simulink model "FDIA_Toolbox"  (R2018a)
settings: Solver=VariableStepAuto  StartTime=0.0  StopTime=10.0  RelTol=1e-3
libraries: commrandsrc3 x30, commutil2 x12, simulink_extras x6, simulink x4, commsynccomp2 x2, commanapbnd3 x2
(part 1 of 2)
settings Model: Creator=sasanka  LastModifiedBy=sasanka

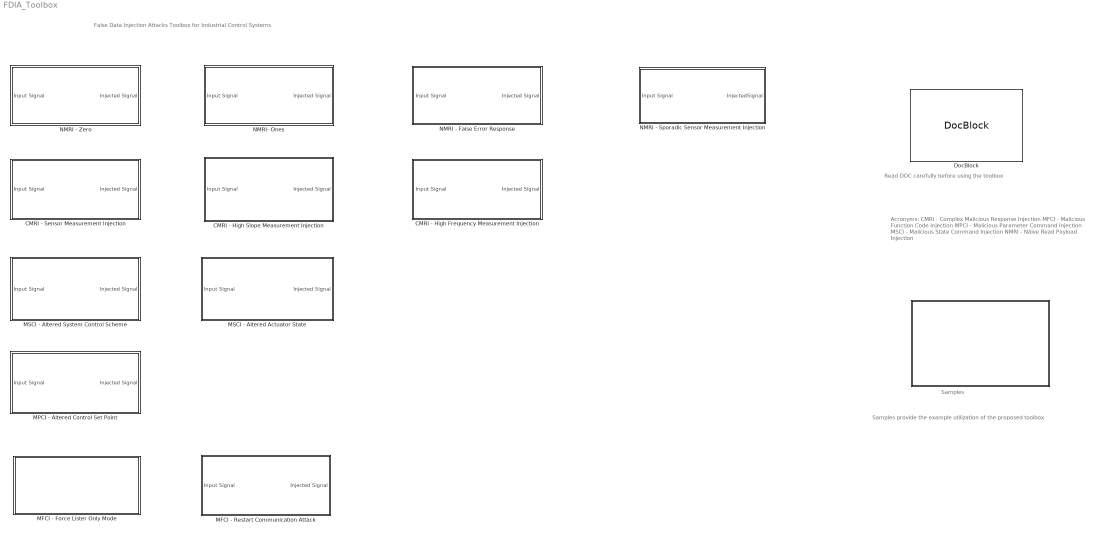
== system FDIA_Toolbox ==
  note: Samples provide the example utilization of the proposed toolbox
  note: Read DOC carefully before using the toolbox
  note: Acronyms:
      |
      | CMRI - Complex Malicious Response Injection
      | MFCI - Malicious Function Code Injection
      | MPCI - Malicious Parameter Command Injection
      | MSCI - Malicious State Command Injection
      | NMRI - Näive Read Payload Injection
  note: False Data Injection Attacks Toolbox for Industrial Control Systems
  note: Samples
  "  " : Subsystem
  CMRI - High Frequency Measurement Injection : Subsystem
  CMRI - High Slope Measurement Injection : Subsystem
  "CMRI - Sensor Measurement Injection " : Subsystem
  DocBlock : simulink/Model-Wide Utilities/DocBlock  DocumentType=Text
      content=|
      | Flase Data Injection Attack (FDIA) Toolbox:
      |
      | People who are using this toolbox are recomended to read the paper "Industrial Contrll System Cyber Attacks" by Thomas H. Morris, Wei Gao
      | Proceedings of the 1st Internatioanl Symposium for ICS & SCADA Cyber Security Research 2013
      |
      | It is found under the following link:
      | https://ewic.bcs.org/upload/pdf/ewic_icscsr13_paper3.pdf (Last Accessed: 19.07.2019)
      |
      | The toolbox is Published under "Development of Injection Attacks Toolbox in MATLAB/Simulnk for Attacks Simulation in Industrial Control System Applications" by Sasanka Potluri, Christian Diedrich, Sai Ram Roy Nanduru and Kishore Vasamshetty
      | in 17th IEEE International Conference on Industrial Informatics INDIN 2019.
      |
      | People who found this library useful for their work are recommend to site the paper.
      |
      | A descrption of the attacks and their impact on the ICS were discussed in the paper in detail.
      |
      | Note: Before using read the paper carefully. The blocks are designed based on some assumtions about a plant.
      |
      | In order to use the block efficiently, you need to change the constants, gains and switching condition according to your plant requirements
      |
      | In some block the properties of the plant needs to be inserted into the block. This will go into the plant moodel block in the toolbox of each attack injection strategy
  "MFCI - Force Lister Only Mode " : Subsystem
  MFCI - Restart Communication Attack : Subsystem
  MPCI - Altered Control Set Point : Subsystem
  MSCI - Altered Actuator State : Subsystem
  "MSCI - Altered System Control Scheme " : Subsystem
  NMRI - False Error Response : Subsystem
  NMRI - Sporadic Sensor Measurement Injection : Subsystem
  NMRI - Zero : Subsystem
  NMRI- Ones : Subsystem  Tag=NMRI - Ones  Description=NMRI - Ones

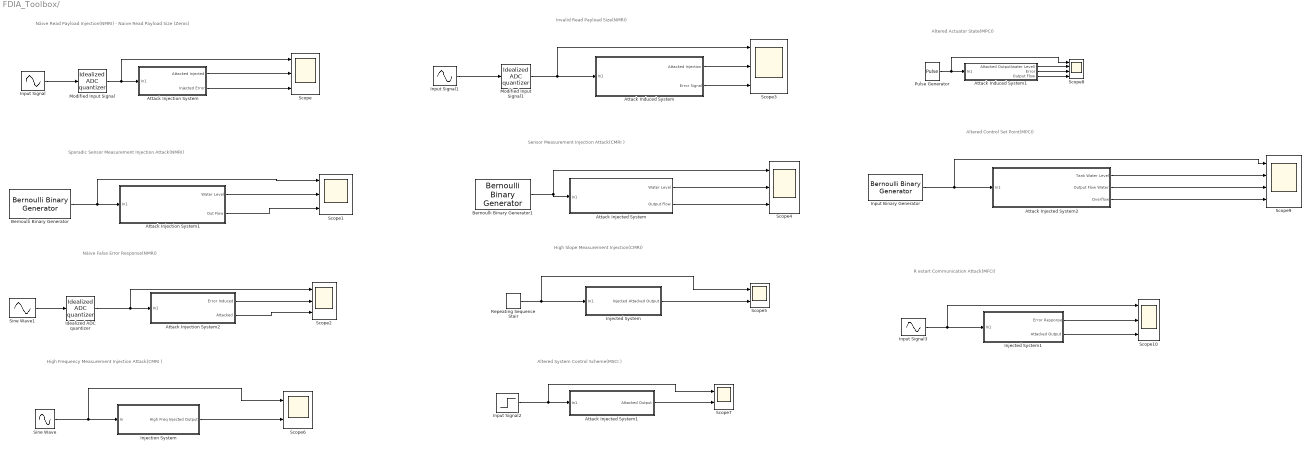
== system FDIA_Toolbox/   ==
  note: Näive Read Payload Injection(NMRI) - Naive Read Payload Size (Zeros)
  note: Sporadic Sensor Measurement Injection Attack(NMRI)
  note: Näive False Error Response(NMRI)
  note: Invalid Read Payload Size(NMRI)
  note: Sensor Measurement Injection Attack(CMRI )
  note: High Slope Measurement Injection(CMRI)
  note: High Frequency Measurement Injection Attack(CMRI )
  note: Altered System Control Scheme(MSCI )
  note: Altered Actuator State(MPCI)
  note: Altered Control Set Point(MPCI)
  note: R estart Communication Attack(MFCI)
  Attack Induced System : Subsystem
  Attack Induced System1 : Subsystem
  Attack Injected System : Subsystem
  Attack Injected System1 : Subsystem
  Attack Injected System2 : Subsystem
  Attack Injection System : Subsystem
  Attack Injection System1 : Subsystem
  Attack Injection System2 : Subsystem
  Bernoulli Binary Generator : commrandsrc3/Bernoulli Binary Generator  ProbabilityOfZero=0.98  SeedSource=Auto  Seed=2  SampleTime=2  SamplesPerFrame=1  OutputDataType=double  SimulateUsing=Interpreted execution
  Bernoulli Binary Generator1 : commrandsrc3/Bernoulli Binary Generator  ProbabilityOfZero=0.9  SeedSource=Auto  Seed=0  SampleTime=15  SamplesPerFrame=1  OutputDataType=double  SimulateUsing=Interpreted execution
  Idealized ADC quantizer : simulink_extras/Additional Discrete/Idealized ADC quantizer  NumberOfConverterBits=8  Vmin=-4  Vmax=16  OutputDataType=uint8  OutputNegativeValues=on
      settings: SourceProductName=Simulink
  Injected System : Subsystem
  Injected System1 : Subsystem
  Injection System : Subsystem
  Input Binary Generator : commrandsrc3/Bernoulli Binary Generator  ProbabilityOfZero=0.98888888  SeedSource=Auto  Seed=2  SampleTime=1  SamplesPerFrame=1  OutputDataType=double  SimulateUsing=Interpreted execution
  Input Signal : Sin  SineType=Sample based  Amplitude=2  Samples=30  SampleTime=1
  Input Signal1 : Sin  SineType=Sample based  Amplitude=2  Samples=30  SampleTime=1
  Input Signal2 : Step  After=1.5
  Input Signal3 : Sin  SineType=Sample based  Amplitude=2  Samples=100  SampleTime=0.5  VectorParams1D=off  Offset=10
  Modified Input Signal : simulink_extras/Additional Discrete/Idealized ADC quantizer  NumberOfConverterBits=8  Vmin=-4  Vmax=16  OutputDataType=uint8  OutputNegativeValues=on
      settings: SourceProductName=Simulink
  Modified Input Signal1 : simulink_extras/Additional Discrete/Idealized ADC quantizer  NumberOfConverterBits=8  Vmin=-4  Vmax=16  OutputDataType=uint8  OutputNegativeValues=on
      settings: SourceProductName=Simulink
  Pulse Generator : DiscretePulseGenerator  Period=15  PulseWidth=10
  Repeating Sequence Stair : simulink/Sources/Repeating Sequence Stair  OutValues="[9 8 7  6 5 4 3 2 1].'"  tsamp=1  OutMin=[]  OutMax=[]  OutDataTypeStr=double  OutputDataTypeScalingMode=double  OutDataType=fixdt(0,8)  ConRadixGroup=Best Precision: Vector-wise  OutScaling=2^-12
      settings: LockScale=on
  Scope{,1..4,10} (6 alike) : Scope  NumInputPorts=3
      Scope10 settings: LoadFcn=plot(ScopeData.time,ScopeData.signals.values)
  Scope5 : Scope  NumInputPorts=2
  Scope6 : Scope  NumInputPorts=2
  Scope7 : Scope  NumInputPorts=2
  Scope8 : Scope  NumInputPorts=4
  Scope9 : Scope  NumInputPorts=4
  Sine Wave : Sin  Frequency=2  SampleTime=0.01
  Sine Wave1 : Sin  SineType=Sample based  Amplitude=2  SampleTime=1
  wires:
  Attack Injection System/2(Injected Error) -> Scope/3
  Modified Input Signal/1 -> Scope/1, Attack Injection System/1(In1)
  Attack Injection System/1(Attacked Injected) -> Scope/2
  Input Signal/1 -> Modified Input Signal/1
  Bernoulli Binary Generator/1 -> Scope1/1, Attack Injection System1/1(In1)
  Attack Injection System1/1(Water Level) -> Scope1/2
  Attack Injection System1/2(Out Flow) -> Scope1/3
  Idealized ADC quantizer/1 -> Scope2/1, Attack Injection System2/1(In1)
  Attack Injection System2/1(Error Induced) -> Scope2/2
  Attack Injection System2/2("Attacked ") -> Scope2/3
  Sine Wave1/1 -> Idealized ADC quantizer/1
  Attack Induced System/2(Error Signal) -> Scope3/3
  Input Signal1/1 -> Modified Input Signal1/1
  Attack Induced System/1(Attacked Injection) -> Scope3/2
  Modified Input Signal1/1 -> Scope3/1, Attack Induced System/1(In1)
  Attack Injected System/2(Output Flow) -> Scope4/3
  Attack Injected System/1(Water Level) -> Scope4/2
  Bernoulli Binary Generator1/1 -> Scope4/1, Attack Injected System/1(In1)
  Repeating Sequence Stair/1 -> Scope5/1, Injected System/1(In1)
  Injected System/1(Injected Attacked Output) -> Scope5/2
  Sine Wave/1 -> Scope6/1, Injection System/1(In)
  Injection System/1(High Freq Injected Output) -> Scope6/2
  Input Signal2/1 -> Scope7/1, Attack Injected System1/1(In1)
  Attack Injected System1/1(Attacked Output) -> Scope7/2
  Attack Induced System1/3(Output Flow) -> Scope8/4
  Attack Induced System1/1(Attacked Output(water Level)) -> Scope8/2
  Pulse Generator/1 -> Scope8/1, Attack Induced System1/1(In1)
  Attack Induced System1/2("Error ") -> Scope8/3
  Attack Injected System2/2(Output Flow Water) -> Scope9/3
  Attack Injected System2/3("Overflow ") -> Scope9/4
  Input Binary Generator/1 -> Scope9/1, Attack Injected System2/1(In1)
  Attack Injected System2/1(Tank Water Level) -> Scope9/2
  Injected System1/2(Attacked Output) -> Scope10/3
  Injected System1/1(Error Response) -> Scope10/2
  Input Signal3/1 -> Scope10/1, Injected System1/1(In1)

== system FDIA_Toolbox/CMRI - High Frequency Measurement Injection ==
  note: Attack Injection Strategy
  Input Signal : Inport
  Add : Sum
  Bernoulli Binary Generator : commrandsrc3/Bernoulli Binary Generator  ProbabilityOfZero=0.82  SeedSource=Auto  Seed=0  SampleTime=1  SamplesPerFrame=1  OutputDataType=double  SimulateUsing=Interpreted execution
  FM Modulator Passband : commanapbnd3/FM Modulator Passband  Fc=5  Ph=0  Kc=3
      settings: SourceProductName=Communications System Toolbox  SourceProductBaseCode=CM
  Logical Operator : Logic  Operator=NOT  AllPortsSameDT=off  OutDataTypeStr=boolean
  Product : Product
  Product1 : Product
  Sine Wave1 : Sin  Frequency=2  SampleTime=0.01
  Injected Signal : Outport
  wires:
  FM Modulator Passband/1 -> Product/1
  Product1/1 -> Add/1
  Logical Operator/1 -> Product1/2
  Add/1 -> Injected Signal/1
  Product/1 -> Add/2
  Bernoulli Binary Generator/1 -> Logical Operator/1, Product/2
  Sine Wave1/1 -> Product1/1
  Input Signal/1 -> FM Modulator Passband/1

== system FDIA_Toolbox/CMRI - High Slope Measurement Injection ==
  note: Attack Injection Strategy
  Input Signal : Inport
  Step : Step  After=0  SampleTime=15
  Step1 : Step  Before=1  After=0  SampleTime=15
  Sum of Elements : Sum  Inputs=+++++++
  Switch : Switch  Criteria=u2 > Threshold
  Transport Delay : TransportDelay  DelayTime=15
  Transport Delay1 : TransportDelay  DelayTime=30
  Transport Delay2 : TransportDelay  DelayTime=45
  Transport Delay3 : TransportDelay  DelayTime=60
  Transport Delay4 : TransportDelay  DelayTime=75
  Transport Delay5 : TransportDelay  DelayTime=90
  Injected Signal : Outport
  wires:
  Transport Delay4/1 -> Sum of Elements/5
  Transport Delay1/1 -> Sum of Elements/2
  Transport Delay2/1 -> Sum of Elements/3
  Sum of Elements/1 -> Injected Signal/1
  Transport Delay/1 -> Sum of Elements/1
  Transport Delay3/1 -> Sum of Elements/4
  Switch/1 -> Transport Delay2/1, Transport Delay3/1, Transport Delay5/1, Transport Delay4/1, Transport Delay1/1, Transport Delay/1, Sum of Elements/6
  Input Signal/1 -> Switch/1
  Step/1 -> Switch/3
  Step1/1 -> Switch/2
  Transport Delay5/1 -> Sum of Elements/7

== system FDIA_Toolbox/CMRI - Sensor Measurement Injection  ==
  note: Attack Injection Strategy
  Input Signal : Inport
  Add1 : Sum
  Bernoulli Binary Generator : commrandsrc3/Bernoulli Binary Generator  ProbabilityOfZero=0.9  SeedSource=Auto  Seed=0  SampleTime=15  SamplesPerFrame=1  OutputDataType=double  SimulateUsing=Interpreted execution
  Logical Operator1 : Logic  Operator=NOT  AllPortsSameDT=off  OutDataTypeStr=boolean
  Plant Model : Subsystem
  Product1 : Product
  Product2 : Product
  Pulse Generator1 : DiscretePulseGenerator  PulseType=Time based  Amplitude=2  Period=15  PulseWidth=65
  Pulse Generator2 : DiscretePulseGenerator  PulseType=Time based  Amplitude=2  Period=20  PulseWidth=75
  Saturation : Saturate  UpperLimit=2  LowerLimit=0
  Injected Signal : Outport
  wires:
  Pulse Generator2/1 -> Product2/2
  Product1/1 -> Add1/1
  Bernoulli Binary Generator/1 -> Product2/1, Logical Operator1/1
  Add1/1 -> Saturation/1
  Product2/1 -> Add1/2
  Logical Operator1/1 -> Product1/2
  Pulse Generator1/1 -> Product1/1
  Saturation/1 -> Plant Model/1(Injection Strategy)
  Input Signal/1 -> Plant Model/2(Input Signal)
  Plant Model/1(Injected Signal) -> Injected Signal/1

== system FDIA_Toolbox/MFCI - Force Lister Only Mode  ==
  note: Edit MATLAB function accordingly to input the plant data and run to code to open the GUI
  MATLAB Function : MATLAB Function  TreatAsAtomicUnit=on

== system FDIA_Toolbox/MFCI - Restart Communication Attack ==
  note: Attack Injection Strategy
  Input Signal : Inport
  Add1 : Sum
  Bernoulli Binary Generator1 : commrandsrc3/Bernoulli Binary Generator  ProbabilityOfZero=0.95  SeedSource=Auto  Seed=0  SampleTime=1  SamplesPerFrame=1  OutputDataType=uint8  SimulateUsing=Interpreted execution
  Constant : Constant  Value=.5  VectorParams1D=off  OutDataTypeStr=uint8
  Logical Operator1 : Logic  Operator=NOT  AllPortsSameDT=off  OutDataTypeStr=boolean
  Product1 : Product
  Product2 : Product
  Injected Signal : Outport
  wires:
  Logical Operator1/1 -> Product1/2
  Constant/1 -> Product2/2
  Add1/1 -> Injected Signal/1
  Product2/1 -> Add1/2
  Bernoulli Binary Generator1/1 -> Product2/1, Logical Operator1/1
  Product1/1 -> Add1/1
  Input Signal/1 -> Product1/1

== system FDIA_Toolbox/MPCI - Altered Control Set Point ==
  note: Attack Injection Strategy
  Input Signal : Inport
  Add1 : Sum
  Bernoulli Binary Generator : commrandsrc3/Bernoulli Binary Generator  ProbabilityOfZero=0.98888888888  SeedSource=Auto  Seed=2  SampleTime=1  SamplesPerFrame=1  OutputDataType=double  SimulateUsing=Interpreted execution
  Input Binary Generator : commrandsrc3/Bernoulli Binary Generator  ProbabilityOfZero=0.98888888  SeedSource=Auto  Seed=2  SampleTime=1  SamplesPerFrame=1  OutputDataType=double  SimulateUsing=Interpreted execution
  Logical Operator1 : Logic  Operator=NOT  AllPortsSameDT=off  OutDataTypeStr=boolean
  Plant Model : Subsystem
  Product1 : Product
  Product2 : Product
  Pulse Generator1 : DiscretePulseGenerator  PulseType=Time based  Amplitude=2  Period=10  PulseWidth=70
  Pulse Generator2 : DiscretePulseGenerator  PulseType=Time based  Amplitude=2  Period=15  PulseWidth=70
  Rate Transition : RateTransition  OutPortSampleTime=0.01
  Saturation : Saturate  UpperLimit=2  LowerLimit=0
  Injected Signal : Outport
  wires:
  Product1/1 -> Add1/1
  Add1/1 -> Saturation/1
  Rate Transition/1 -> Logical Operator1/1
  Pulse Generator1/1 -> Product1/1
  Logical Operator1/1 -> Product1/2
  Product2/1 -> Add1/2
  Pulse Generator2/1 -> Product2/2
  Bernoulli Binary Generator/1 -> Product2/1
  Input Binary Generator/1 -> Rate Transition/1
  Plant Model/1(Injected Signal) -> Injected Signal/1
  Saturation/1 -> Plant Model/1(Injection Strategy)
  Input Signal/1 -> Plant Model/2(Input Signal)

== system FDIA_Toolbox/MSCI - Altered Actuator State ==
  note: Attack Injection Strategy
  Input Signal : Inport
  Bernoulli Binary Generator2 : commrandsrc3/Bernoulli Binary Generator  ProbabilityOfZero=0.6  SeedSource=Auto  Seed=0  SampleTime=1  SamplesPerFrame=1  OutputDataType=double  SimulateUsing=Interpreted execution
  Plant Model : Subsystem
  Product2 : Product
  Pulse Generator : DiscretePulseGenerator  Period=15  PulseWidth=10
  Injected Signal : Outport
  wires:
  Bernoulli Binary Generator2/1 -> Product2/2
  Plant Model/1(Injected Signal) -> Injected Signal/1
  Product2/1 -> Plant Model/1(Injection Strategy)
  Input Signal/1 -> Plant Model/2(Input Signal)
  Pulse Generator/1 -> Product2/1

== system FDIA_Toolbox/MSCI - Altered System Control Scheme  ==
  note: Attack Injection Strategy
  Input Signal : Inport
  Add : Sum  Inputs=+++
  Add2 : Sum  Inputs=+-
  Derivative : Derivative
  Gain : Gain  Gain=5
  Gain1 : Gain  Gain=15
  Gain2 : Gain  Gain=10
  Integrator : Integrator  InitialCondition=1
  Manual Signal : Subsystem
  Step3 : Step  Time=50
  Switch : Switch  Criteria=u2 > Threshold
  Transfer Fcn : TransferFcn  Denominator=[1 0.5 0.1]  ContinuousStateAttributes='position'
  Injected Signal : Outport
  wires:
  Step3/1 -> Switch/2
  Add2/1 -> Gain/1, Gain2/1, Gain1/1
  Gain1/1 -> Integrator/1
  Derivative/1 -> Add/3
  Gain/1 -> Add/1
  Transfer Fcn/1 -> Injected Signal/1, Add2/2, Manual Signal/1(In1)  "y(t)"
  Input Signal/1 -> Add2/1
  Switch/1 -> Transfer Fcn/1
  Integrator/1 -> Add/2
  Gain2/1 -> Derivative/1
  Add/1 -> Switch/3
  Manual Signal/1(Out1) -> Switch/1

== system FDIA_Toolbox/NMRI - False Error Response ==
  Input Signal : Inport
  Attack Injection Strategy : Subsystem
  Idealized ADC quantizer : simulink_extras/Additional Discrete/Idealized ADC quantizer  NumberOfConverterBits=8  Vmin=-4  Vmax=16  OutputDataType=uint8  OutputNegativeValues=on
      settings: SourceProductName=Simulink
  Injected Signal : Outport
  wires:
  Attack Injection Strategy/2("Attacked ") -> Injected Signal/1
  Input Signal/1 -> Idealized ADC quantizer/1
  Idealized ADC quantizer/1 -> Attack Injection Strategy/1(In1)

== system FDIA_Toolbox/NMRI - Sporadic Sensor Measurement Injection ==
  note: Attack Injection Strategy
  Input Signal : Inport
  Add1 : Sum
  Bernoulli Binary Generator : commrandsrc3/Bernoulli Binary Generator  ProbabilityOfZero=0.98  SeedSource=Auto  Seed=2  SampleTime=2  SamplesPerFrame=1  OutputDataType=double  SimulateUsing=Interpreted execution
  Logical Operator1 : Logic  Operator=NOT  AllPortsSameDT=off  OutDataTypeStr=boolean
  Plant Model : Subsystem
  Product1 : Product  RndMeth=Nearest
  Product2 : Product
  Pulse Generator1 : DiscretePulseGenerator  PulseType=Time based  Amplitude=2  Period=10  PulseWidth=70
  Pulse Generator4 : DiscretePulseGenerator  PulseType=Time based  Amplitude=2  PulseWidth=52
  Rate Transition : RateTransition
  Saturation : Saturate  UpperLimit=2  LowerLimit=0
  InjectedSignal : Outport
  wires:
  Product2/1 -> Add1/2
  Product1/1 -> Add1/1
  Bernoulli Binary Generator/1 -> Product2/1, Rate Transition/1
  Pulse Generator4/1 -> Product2/2
  Logical Operator1/1 -> Product1/2
  Pulse Generator1/1 -> Product1/1
  Add1/1 -> Saturation/1
  Rate Transition/1 -> Logical Operator1/1
  Saturation/1 -> Plant Model/1(Injection Strategy)
  Input Signal/1 -> Plant Model/2(Input Signal)
  Plant Model/1(Injected Signal) -> InjectedSignal/1

== system FDIA_Toolbox/NMRI - Zero ==
  Input Signal : Inport
  Attack Injection Strategy : Subsystem
  Modified Input Signal : simulink_extras/Additional Discrete/Idealized ADC quantizer  NumberOfConverterBits=8  Vmin=-4  Vmax=16  OutputDataType=uint8  OutputNegativeValues=on
      settings: SourceProductName=Simulink
  Injected Signal : Outport
  wires:
  Attack Injection Strategy/1(Injected Signal) -> Injected Signal/1
  Modified Input Signal/1 -> Attack Injection Strategy/1(Input)
  Input Signal/1 -> Modified Input Signal/1

== system FDIA_Toolbox/NMRI- Ones ==
  Input Signal : Inport
  Attack Induced Strategy : Subsystem
  Modified Input Signal : simulink_extras/Additional Discrete/Idealized ADC quantizer  NumberOfConverterBits=8  Vmin=-4  Vmax=16  OutputDataType=uint8  OutputNegativeValues=on
      settings: SourceProductName=Simulink
  Injected Signal : Outport
  wires:
  Modified Input Signal/1 -> Attack Induced Strategy/1(In1)
  Attack Induced Strategy/1(Attacked Injection) -> Injected Signal/1
  Input Signal/1 -> Modified Input Signal/1

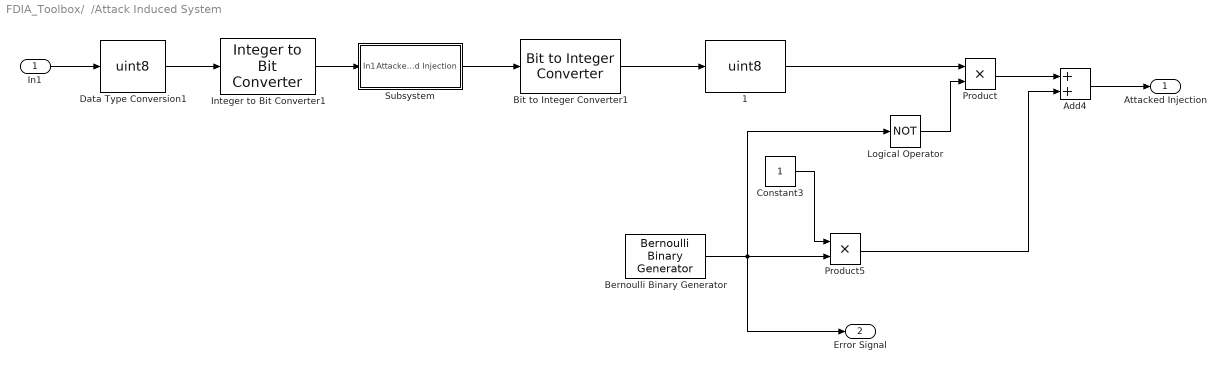
== system FDIA_Toolbox/  /Attack Induced System ==
  In1 : Inport
  " 1" : DataTypeConversion  OutMin=15  OutMax=16  OutDataTypeStr=uint8  ConvertRealWorld=Stored Integer (SI)  RndMeth=Round  SaturateOnIntegerOverflow=on  LockScale=on
  Add4 : Sum
  Bernoulli Binary Generator : commrandsrc3/Bernoulli Binary Generator  ProbabilityOfZero=0.9  SeedSource=Auto  Seed=0  SampleTime=1  SamplesPerFrame=1  OutputDataType=boolean  SimulateUsing=Interpreted execution
  Bit to Integer Converter1 : commutil2/Bit to Integer Converter  nbits=32  bitOrder=MSB first  signedOutputValues=Unsigned  outDtype=uint8  outDtypeSigned=int8
  Constant3 : Constant  OutDataTypeStr=boolean
  Data Type Conversion1 : DataTypeConversion  OutMin=15  OutMax=16  OutDataTypeStr=uint8  ConvertRealWorld=Stored Integer (SI)  RndMeth=Round  SaturateOnIntegerOverflow=on  LockScale=on
  Integer to Bit Converter1 : commutil2/Integer to Bit Converter  nbits=32  signedInputValues=Unsigned  bitOrder=MSB first  outDtype=uint8
  Logical Operator : Logic  Operator=NOT  AllPortsSameDT=off  OutDataTypeStr=boolean
  Product : Product  OutDataTypeStr=uint8
  Product5 : Product  OutDataTypeStr=uint8
  Subsystem : Subsystem
  Attacked Injection : Outport
  Error Signal : Outport  Port=2
  wires:
  In1/1 -> Data Type Conversion1/1
  Bernoulli Binary Generator/1 -> Error Signal/1, Logical Operator/1, Product5/2
  Bit to Integer Converter1/1 -> " 1"/1
  Subsystem/1(Attacked Injection) -> Bit to Integer Converter1/1
  Integer to Bit Converter1/1 -> Subsystem/1(In1)
  Data Type Conversion1/1 -> Integer to Bit Converter1/1
  Constant3/1 -> Product5/1
  " 1"/1 -> Product/1
  Logical Operator/1 -> Product/2
  Add4/1 -> Attacked Injection/1
  Product/1 -> Add4/1
  Product5/1 -> Add4/2

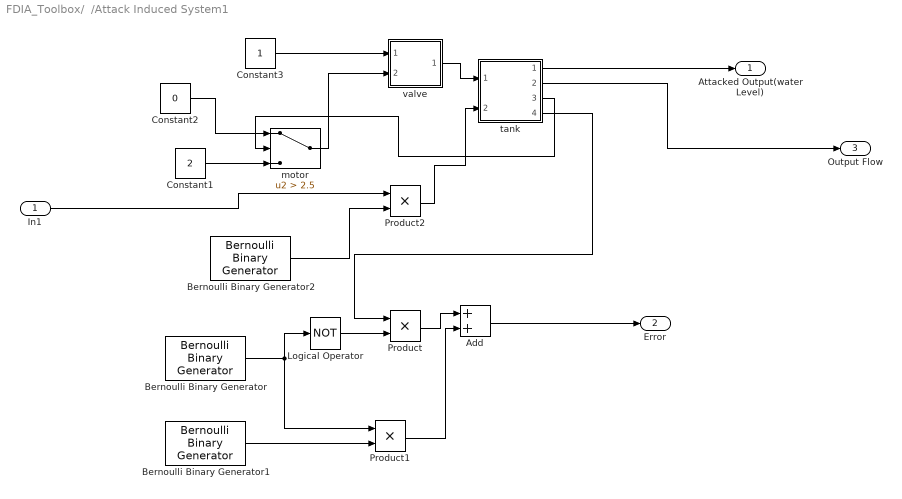
== system FDIA_Toolbox/  /Attack Induced System1 ==
  In1 : Inport
  Add : Sum
  Bernoulli Binary Generator : commrandsrc3/Bernoulli Binary Generator  ProbabilityOfZero=0.9  SeedSource=Auto  Seed=0  SampleTime=1  SamplesPerFrame=1  OutputDataType=double  SimulateUsing=Interpreted execution
  Bernoulli Binary Generator1 : commrandsrc3/Bernoulli Binary Generator  ProbabilityOfZero=0.9  SeedSource=Auto  Seed=0  SampleTime=1  SamplesPerFrame=1  OutputDataType=double  SimulateUsing=Interpreted execution
  Bernoulli Binary Generator2 : commrandsrc3/Bernoulli Binary Generator  ProbabilityOfZero=0.6  SeedSource=Auto  Seed=0  SampleTime=1  SamplesPerFrame=1  OutputDataType=double  SimulateUsing=Interpreted execution
  Constant1 : Constant  Value=2  SampleTime=1
  Constant2 : Constant  Value=0  SampleTime=1
  Constant3 : Constant  SampleTime=1
  Logical Operator : Logic  Operator=NOT  AllPortsSameDT=off  OutDataTypeStr=boolean
  Product : Product
  Product1 : Product
  Product2 : Product
  "motor " : Switch  Criteria=u2 > Threshold  Threshold=2.5  ZeroCross=off
  "tank " : Subsystem  mask(Water tank){ht=15, area=1, outletArea=0.1, overflowLimit=4, initialHt=0}
      mask prompts: ht "Height of tank (m):"; area "Bottom area (m^2):"; outletArea "Out pipe crossection (m^2):"; overflowLimit "Overflow sensor distance from top (m):"; initialHt "Initial level height (m):"
      mask help: Cylindrical water tank with overflow signal
      mask Display: disp('WATER\nTANK')
  valve : Subsystem  mask(Valve){InitialPosition=0}
      mask prompts: InitialPosition "Initial position [0=closed 1=open]:"
      mask help: Valve
      mask Display: disp('VALVE')
  Attacked Output(water Level) : Outport
  "Error " : Outport  Port=2
  Output Flow : Outport  Port=3
  wires:
  Add/1 -> "Error "/1
  Constant1/1 -> "motor "/3
  "tank "/4(water level1) -> Product/1
  Product/1 -> Add/1
  "tank "/1(water level) -> Attacked Output(water Level)/1
  "motor "/1 -> valve/2(source flow)
  Product1/1 -> Add/2
  Constant3/1 -> valve/1(control)
  valve/1(out flow) -> "tank "/1(flow in)
  Constant2/1 -> "motor "/1
  Bernoulli Binary Generator/1 -> Logical Operator/1, Product1/1
  Logical Operator/1 -> Product/2
  Bernoulli Binary Generator1/1 -> Product1/2
  Product2/1 -> "tank "/2(flow in1)
  "tank "/3(overflow flag) -> "motor "/2
  Bernoulli Binary Generator2/1 -> Product2/2
  In1/1 -> Product2/1
  "tank "/2(flow out) -> Output Flow/1

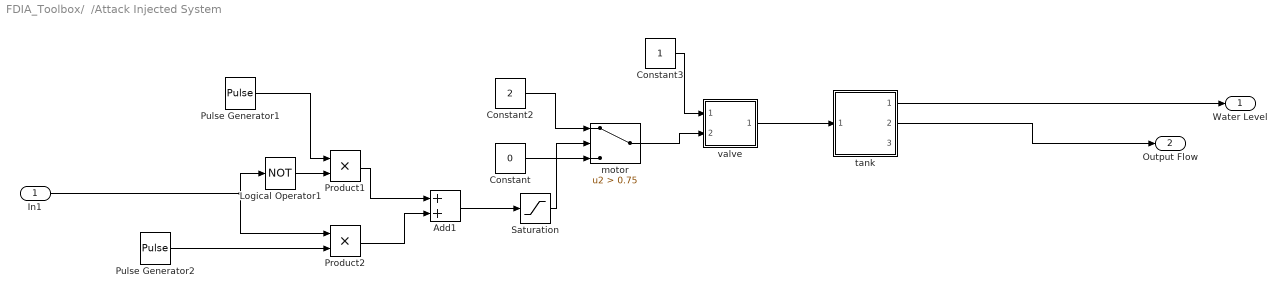
== system FDIA_Toolbox/  /Attack Injected System ==
  In1 : Inport
  Add1 : Sum
  Constant : Constant  Value=0
  Constant2 : Constant  Value=2
  Constant3 : Constant
  Logical Operator1 : Logic  Operator=NOT  AllPortsSameDT=off  OutDataTypeStr=boolean
  Product1 : Product
  Product2 : Product
  Pulse Generator1 : DiscretePulseGenerator  PulseType=Time based  Amplitude=2  Period=15  PulseWidth=65
  Pulse Generator2 : DiscretePulseGenerator  PulseType=Time based  Amplitude=2  Period=20  PulseWidth=75
  Saturation : Saturate  UpperLimit=2  LowerLimit=0
  "motor " : Switch  Criteria=u2 > Threshold  Threshold=0.75  ZeroCross=off
  "tank " : Subsystem  mask(Water tank){ht=15, area=1, outletArea=0.1, overflowLimit=0, initialHt=0}
      mask prompts: ht "Height of tank (m):"; area "Bottom area (m^2):"; outletArea "Out pipe crossection (m^2):"; overflowLimit "Overflow sensor distance from top (m):"; initialHt "Initial level height (m):"
      mask help: Cylindrical water tank with overflow signal
      mask Display: disp('WATER\nTANK')
  valve : Subsystem  mask(Valve){InitialPosition=0}
      mask prompts: InitialPosition "Initial position [0=closed 1=open]:"
      mask help: Valve
      mask Display: disp('VALVE')
  Water Level : Outport
  Output Flow : Outport  Port=2
  wires:
  "tank "/1(water level) -> Water Level/1
  "motor "/1 -> valve/2(source flow)
  Add1/1 -> Saturation/1
  Constant3/1 -> valve/1(control)
  Pulse Generator1/1 -> Product1/1
  valve/1(out flow) -> "tank "/1(flow in)
  Constant2/1 -> "motor "/1
  Constant/1 -> "motor "/3
  Logical Operator1/1 -> Product1/2
  Product1/1 -> Add1/1
  Pulse Generator2/1 -> Product2/2
  Product2/1 -> Add1/2
  Saturation/1 -> "motor "/2
  In1/1 -> Product2/1, Logical Operator1/1
  "tank "/2(flow out) -> Output Flow/1

== system FDIA_Toolbox/  /Attack Injected System1 ==
  In1 : Inport
  Add : Sum  Inputs=+++
  Add2 : Sum  Inputs=+-
  Derivative : Derivative
  Gain : Gain  Gain=5
  Gain1 : Gain  Gain=15
  Gain2 : Gain  Gain=10
  Integrator : Integrator  InitialCondition=1
  Manual Signal : Subsystem
  Step3 : Step  Time=50
  Switch : Switch  Criteria=u2 > Threshold
  Transfer Fcn : TransferFcn  Denominator=[1 0.5 0.1]  ContinuousStateAttributes='position'
  Attacked Output : Outport
  wires:
  Step3/1 -> Switch/2
  Add2/1 -> Gain/1, Gain2/1, Gain1/1
  Gain1/1 -> Integrator/1
  Derivative/1 -> Add/3
  Gain/1 -> Add/1
  Transfer Fcn/1 -> Attacked Output/1, Add2/2, Manual Signal/1(In1)  "y(t)"
  In1/1 -> Add2/1
  Switch/1 -> Transfer Fcn/1
  Integrator/1 -> Add/2
  Gain2/1 -> Derivative/1
  Add/1 -> Switch/3
  Manual Signal/1(Out1) -> Switch/1

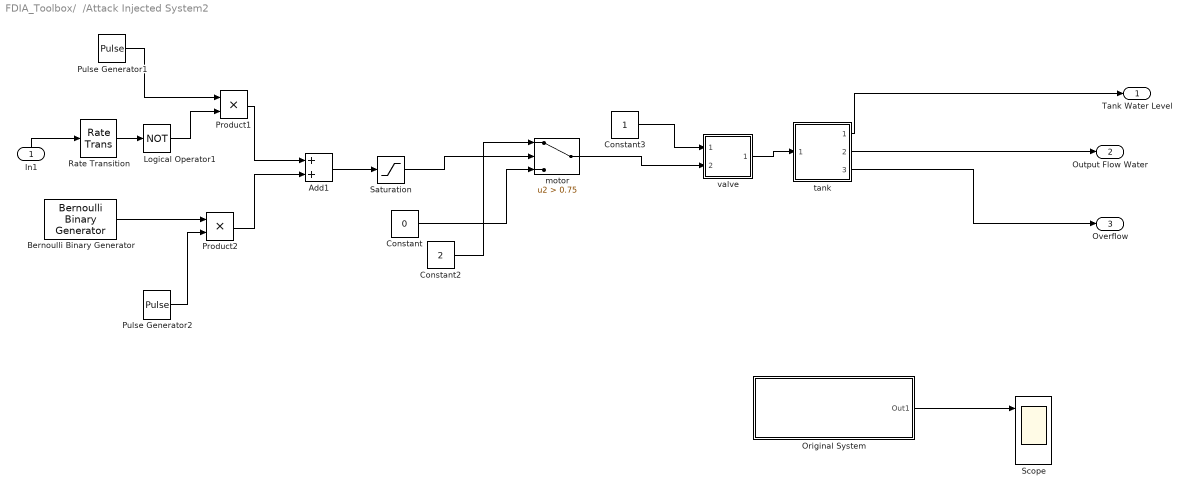
== system FDIA_Toolbox/  /Attack Injected System2 ==
  In1 : Inport
  Add1 : Sum
  Bernoulli Binary Generator : commrandsrc3/Bernoulli Binary Generator  ProbabilityOfZero=0.98888888888  SeedSource=Auto  Seed=2  SampleTime=1  SamplesPerFrame=1  OutputDataType=double  SimulateUsing=Interpreted execution
  Constant : Constant  Value=0
  Constant2 : Constant  Value=2
  Constant3 : Constant
  Logical Operator1 : Logic  Operator=NOT  AllPortsSameDT=off  OutDataTypeStr=boolean
  Original System : Subsystem
  Product1 : Product
  Product2 : Product
  Pulse Generator1 : DiscretePulseGenerator  PulseType=Time based  Amplitude=2  Period=10  PulseWidth=70
  Pulse Generator2 : DiscretePulseGenerator  PulseType=Time based  Amplitude=2  Period=15  PulseWidth=70
  Rate Transition : RateTransition  OutPortSampleTime=0.01
  Saturation : Saturate  UpperLimit=2  LowerLimit=0
  Scope : Scope  NumInputPorts=3
  "motor " : Switch  Criteria=u2 > Threshold  Threshold=0.75  ZeroCross=off
  "tank " : Subsystem  mask(Water tank){ht=15, area=1, outletArea=0.1, overflowLimit=0, initialHt=0}
      mask prompts: ht "Height of tank (m):"; area "Bottom area (m^2):"; outletArea "Out pipe crossection (m^2):"; overflowLimit "Overflow sensor distance from top (m):"; initialHt "Initial level height (m):"
      mask help: Cylindrical water tank with overflow signal
      mask Display: disp('WATER\nTANK')
  valve : Subsystem  mask(Valve){InitialPosition=0}
      mask prompts: InitialPosition "Initial position [0=closed 1=open]:"
      mask help: Valve
      mask Display: disp('VALVE')
  Tank Water Level : Outport
  Output Flow Water : Outport  Port=2
  "Overflow " : Outport  Port=3
  wires:
  Constant/1 -> "motor "/3
  Constant2/1 -> "motor "/1
  Saturation/1 -> "motor "/2
  Product1/1 -> Add1/1
  Add1/1 -> Saturation/1
  Rate Transition/1 -> Logical Operator1/1
  Pulse Generator1/1 -> Product1/1
  Logical Operator1/1 -> Product1/2
  Product2/1 -> Add1/2
  Pulse Generator2/1 -> Product2/2
  "tank "/1(water level) -> Tank Water Level/1
  Constant3/1 -> valve/1(control)
  "motor "/1 -> valve/2(source flow)
  valve/1(out flow) -> "tank "/1(flow in)
  In1/1 -> Rate Transition/1
  "tank "/2(flow out) -> Output Flow Water/1
  "tank "/3(overflow flag1) -> "Overflow "/1
  Bernoulli Binary Generator/1 -> Product2/1
  Original System/1(Out1) -> Scope/1

== system FDIA_Toolbox/  /Attack Injection System ==
  In1 : Inport
  " 1" : DataTypeConversion  OutMin=15  OutMax=16  OutDataTypeStr=uint8  ConvertRealWorld=Stored Integer (SI)  RndMeth=Round  SaturateOnIntegerOverflow=on  LockScale=on
  Bit to Integer Converter2 : commutil2/Bit to Integer Converter  nbits=32  bitOrder=MSB first  signedOutputValues=Unsigned  outDtype=uint8  outDtypeSigned=int8
  Data Type Conversion2 : DataTypeConversion  OutMin=15  OutMax=16  OutDataTypeStr=uint8  ConvertRealWorld=Stored Integer (SI)  RndMeth=Round  SaturateOnIntegerOverflow=on  LockScale=on
  Integer to Bit Converter : commutil2/Integer to Bit Converter  nbits=32  signedInputValues=Unsigned  bitOrder=MSB first  outDtype=uint8
  Subsystem : Subsystem
  Attacked Injected : Outport
  Injected Error : Outport  Port=2
  wires:
  " 1"/1 -> Attacked Injected/1
  Data Type Conversion2/1 -> Integer to Bit Converter/1
  Integer to Bit Converter/1 -> Subsystem/1(In1)
  Bit to Integer Converter2/1 -> " 1"/1
  Subsystem/1(Attacked) -> Bit to Integer Converter2/1
  Subsystem/2(Injected Error) -> Injected Error/1
  In1/1 -> Data Type Conversion2/1

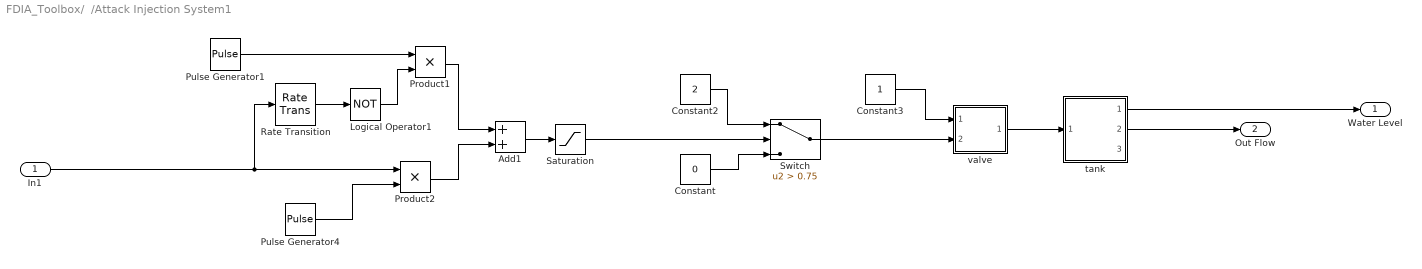
== system FDIA_Toolbox/  /Attack Injection System1 ==
  In1 : Inport
  Add1 : Sum
  Constant : Constant  Value=0
  Constant2 : Constant  Value=2
  Constant3 : Constant
  Logical Operator1 : Logic  Operator=NOT  AllPortsSameDT=off  OutDataTypeStr=boolean
  Product1 : Product  RndMeth=Nearest
  Product2 : Product
  Pulse Generator1 : DiscretePulseGenerator  PulseType=Time based  Amplitude=2  Period=10  PulseWidth=70
  Pulse Generator4 : DiscretePulseGenerator  PulseType=Time based  Amplitude=2  PulseWidth=52
  Rate Transition : RateTransition
  Saturation : Saturate  UpperLimit=2  LowerLimit=0
  "Switch " : Switch  Criteria=u2 > Threshold  Threshold=0.75  ZeroCross=off
  "tank " : Subsystem  mask(Water tank){ht=15, area=1, outletArea=0.1, overflowLimit=0, initialHt=0}
      mask prompts: ht "Height of tank (m):"; area "Bottom area (m^2):"; outletArea "Out pipe crossection (m^2):"; overflowLimit "Overflow sensor distance from top (m):"; initialHt "Initial level height (m):"
      mask help: Cylindrical water tank with overflow signal
      mask Display: disp('WATER\nTANK')
  valve : Subsystem  mask(Valve){InitialPosition=0}
      mask prompts: InitialPosition "Initial position [0=closed 1=open]:"
      mask help: Valve
      mask Display: disp('VALVE')
  Water Level : Outport
  Out Flow : Outport  Port=2
  wires:
  Product1/1 -> Add1/1
  Product2/1 -> Add1/2
  Pulse Generator1/1 -> Product1/1
  Saturation/1 -> "Switch "/2
  In1/1 -> Rate Transition/1, Product2/1
  Rate Transition/1 -> Logical Operator1/1
  Pulse Generator4/1 -> Product2/2
  "tank "/1(water level) -> Water Level/1
  "Switch "/1 -> valve/2(source flow)
  Constant2/1 -> "Switch "/1
  Logical Operator1/1 -> Product1/2
  Add1/1 -> Saturation/1
  valve/1(out flow) -> "tank "/1(flow in)
  Constant/1 -> "Switch "/3
  Constant3/1 -> valve/1(control)
  "tank "/2(flow out) -> Out Flow/1

== system FDIA_Toolbox/  /Attack Injection System2 ==
  In1 : Inport
  " 1" : DataTypeConversion  OutMin=15  OutMax=16  OutDataTypeStr=uint8  ConvertRealWorld=Stored Integer (SI)  RndMeth=Round  SaturateOnIntegerOverflow=on  LockScale=on
  Bit to Integer Converter2 : commutil2/Bit to Integer Converter  nbits=32  bitOrder=MSB first  signedOutputValues=Unsigned  outDtype=uint8  outDtypeSigned=int8
  Data Type Conversion2 : DataTypeConversion  OutMin=15  OutMax=16  OutDataTypeStr=fixdt(1,16)  ConvertRealWorld=Stored Integer (SI)  RndMeth=Round  SaturateOnIntegerOverflow=on  LockScale=on
  Integer to Bit Converter : commutil2/Integer to Bit Converter  nbits=32  signedInputValues=Unsigned  bitOrder=MSB first  outDtype=uint8
  Subsystem : Subsystem
  Error Induced : Outport
  "Attacked " : Outport  Port=2
  wires:
  Data Type Conversion2/1 -> Integer to Bit Converter/1
  Subsystem/1(Output) -> Bit to Integer Converter2/1
  Subsystem/2(Error) -> Error Induced/1
  " 1"/1 -> "Attacked "/1
  In1/1 -> Data Type Conversion2/1
  Bit to Integer Converter2/1 -> " 1"/1
  Integer to Bit Converter/1 -> Subsystem/1(In1)

== system FDIA_Toolbox/  /Injected System ==
  In1 : Inport
  Step : Step  After=0  SampleTime=15
  Step1 : Step  Before=1  After=0  SampleTime=15
  Sum of Elements : Sum  Inputs=+++++++
  Switch : Switch  Criteria=u2 > Threshold
  Transport Delay : TransportDelay  DelayTime=15
  Transport Delay1 : TransportDelay  DelayTime=30
  Transport Delay2 : TransportDelay  DelayTime=45
  Transport Delay3 : TransportDelay  DelayTime=60
  Transport Delay4 : TransportDelay  DelayTime=75
  Transport Delay5 : TransportDelay  DelayTime=90
  Injected Attacked Output : Outport
  wires:
  Transport Delay4/1 -> Sum of Elements/5
  Transport Delay1/1 -> Sum of Elements/2
  Transport Delay2/1 -> Sum of Elements/3
  Sum of Elements/1 -> Injected Attacked Output/1
  Transport Delay/1 -> Sum of Elements/1
  Transport Delay3/1 -> Sum of Elements/4
  Switch/1 -> Transport Delay2/1, Transport Delay3/1, Transport Delay5/1, Transport Delay4/1, Transport Delay1/1, Transport Delay/1, Sum of Elements/6
  In1/1 -> Switch/1
  Step/1 -> Switch/3
  Step1/1 -> Switch/2
  Transport Delay5/1 -> Sum of Elements/7

== system FDIA_Toolbox/  /Injected System1 ==
  In1 : Inport
  Add1 : Sum
  Bernoulli Binary Generator1 : commrandsrc3/Bernoulli Binary Generator  ProbabilityOfZero=0.95  SeedSource=Auto  Seed=0  SampleTime=1  SamplesPerFrame=1  OutputDataType=uint8  SimulateUsing=Interpreted execution
  Constant : Constant  Value=.5  VectorParams1D=off  OutDataTypeStr=uint8
  Demux : Demux  Outputs=1
  Demux1 : Demux  Outputs=1
  Logical Operator1 : Logic  Operator=NOT  AllPortsSameDT=off  OutDataTypeStr=boolean
  Product1 : Product
  Product2 : Product
  Scope1 : Scope
      settings: LoadFcn=plot(ScopeData.time,ScopeData.signals.values)
  Scope2 : Scope
      settings: LoadFcn=plot(ScopeData.time,ScopeData.signals.values)
  Error Response : Outport
  Attacked Output : Outport  Port=2
  wires:
  Logical Operator1/1 -> Product1/2
  Constant/1 -> Product2/2
  Add1/1 -> Attacked Output/1, Demux/1
  Product2/1 -> Demux1/1, Add1/2
  Demux1/1 -> Scope2/1
  Demux/1 -> Scope1/1
  Bernoulli Binary Generator1/1 -> Product2/1, Error Response/1, Logical Operator1/1
  Product1/1 -> Add1/1
  In1/1 -> Product1/1

== system FDIA_Toolbox/  /Injection System ==
  In : Inport
  Add : Sum
  Bernoulli Binary Generator : commrandsrc3/Bernoulli Binary Generator  ProbabilityOfZero=0.82  SeedSource=Auto  Seed=0  SampleTime=1  SamplesPerFrame=1  OutputDataType=double  SimulateUsing=Interpreted execution
  FM Modulator Passband : commanapbnd3/FM Modulator Passband  Fc=5  Ph=0  Kc=3
      settings: SourceProductName=Communications System Toolbox  SourceProductBaseCode=CM
  Logical Operator : Logic  Operator=NOT  AllPortsSameDT=off  OutDataTypeStr=boolean
  Product : Product
  Product1 : Product
  Sine Wave1 : Sin  Frequency=2  SampleTime=0.01
  High Freq Injected Output : Outport
  wires:
  FM Modulator Passband/1 -> Product/1
  Product1/1 -> Add/1
  Logical Operator/1 -> Product1/2
  Add/1 -> High Freq Injected Output/1
  Product/1 -> Add/2
  Bernoulli Binary Generator/1 -> Logical Operator/1, Product/2
  Sine Wave1/1 -> Product1/1
  In/1 -> FM Modulator Passband/1

== system FDIA_Toolbox/CMRI - Sensor Measurement Injection /Plant Model ==
  note: Change product block with you plant mode l
  note: Change the constant values according to the plant requirements
  Injection Strategy : Inport
  Input Signal : Inport  Port=2
  Constant : Constant  Value=0
  Constant2 : Constant  Value=2
  Product : Product
  "motor " : Switch  Criteria=u2 > Threshold  Threshold=0.75  ZeroCross=off
  Injected Signal : Outport
  wires:
  Constant2/1 -> "motor "/1
  Injection Strategy/1 -> "motor "/2
  Constant/1 -> "motor "/3
  "motor "/1 -> Product/1
  Input Signal/1 -> Product/2
  Product/1 -> Injected Signal/1

== system FDIA_Toolbox/MPCI - Altered Control Set Point/Plant Model ==
  note: Change product block with you plant mode l
  note: Change the constant values according to the plant requirements
  Injection Strategy : Inport
  Input Signal : Inport  Port=2
  Constant : Constant  Value=0
  Constant2 : Constant  Value=2
  Product : Product
  "Switch " : Switch  Criteria=u2 > Threshold  Threshold=0.75  ZeroCross=off
  Injected Signal : Outport
  wires:
  Constant/1 -> "Switch "/3
  "Switch "/1 -> Product/1
  Injection Strategy/1 -> "Switch "/2
  Constant2/1 -> "Switch "/1
  Input Signal/1 -> Product/2
  Product/1 -> Injected Signal/1

== system FDIA_Toolbox/MSCI - Altered Actuator State/Plant Model ==
  note: Change product block with you plant mode l
  note: Change the constant values according to the plant requirements
  Injection Strategy : Inport
  Input Signal : Inport  Port=2
  Constant : Constant  Value=0
  Constant2 : Constant  Value=2
  Product : Product
  "Switch " : Switch  Criteria=u2 > Threshold  Threshold=0.75  ZeroCross=off
  Injected Signal : Outport
  wires:
  "Switch "/1 -> Product/1
  Input Signal/1 -> Product/2
  Constant2/1 -> "Switch "/1
  Product/1 -> Injected Signal/1
  Constant/1 -> "Switch "/3
  Injection Strategy/1 -> "Switch "/2

== system FDIA_Toolbox/MSCI - Altered System Control Scheme /Manual Signal ==
  In1 : Inport
  Add1 : Sum  Inputs=+-
  Add3 : Sum
  Continuous-Time VCO : commsynccomp2/Continuous-Time VCO  Ac=0.1  Fc=5  Kc=1  Ph=0
      settings: SourceProductName=Communications System Toolbox  SourceProductBaseCode=CM
  Repeating Sequence Stair : simulink/Sources/Repeating Sequence Stair  OutValues=[0.9 1 1 0.9].'  tsamp=2  OutMin=[]  OutMax=[]  OutDataTypeStr=double  OutputDataTypeScalingMode=double  OutDataType=fixdt(0,8)  ConRadixGroup=Best Precision: Vector-wise  OutScaling=2^-12
  Sine Wave1 : Sin  SineType=Sample based  Amplitude=0.1  Frequency=10  Samples=1000  SampleTime=0.01
  Out1 : Outport
  wires:
  Add3/1 -> Add1/1
  Repeating Sequence Stair/1 -> Add3/1
  Sine Wave1/1 -> Continuous-Time VCO/1
  Continuous-Time VCO/1 -> Add3/2
  Add1/1 -> Out1/1
  In1/1 -> Add1/2

== system FDIA_Toolbox/NMRI - False Error Response/Attack Injection Strategy ==
  In1 : Inport
  " 1" : DataTypeConversion  OutMin=15  OutMax=16  OutDataTypeStr=uint8  ConvertRealWorld=Stored Integer (SI)  RndMeth=Round  SaturateOnIntegerOverflow=on  LockScale=on
  Bit to Integer Converter2 : commutil2/Bit to Integer Converter  nbits=32  bitOrder=MSB first  signedOutputValues=Unsigned  outDtype=uint8  outDtypeSigned=int8
  Data Type Conversion2 : DataTypeConversion  OutMin=15  OutMax=16  OutDataTypeStr=fixdt(1,16)  ConvertRealWorld=Stored Integer (SI)  RndMeth=Round  SaturateOnIntegerOverflow=on  LockScale=on
  Integer to Bit Converter : commutil2/Integer to Bit Converter  nbits=32  signedInputValues=Unsigned  bitOrder=MSB first  outDtype=uint8
  Subsystem : Subsystem
  Error Induced : Outport
  "Attacked " : Outport  Port=2
  wires:
  Data Type Conversion2/1 -> Integer to Bit Converter/1
  Subsystem/1(Output) -> Bit to Integer Converter2/1
  Subsystem/2(Error) -> Error Induced/1
  " 1"/1 -> "Attacked "/1
  In1/1 -> Data Type Conversion2/1
  Bit to Integer Converter2/1 -> " 1"/1
  Integer to Bit Converter/1 -> Subsystem/1(In1)

== system FDIA_Toolbox/NMRI - Sporadic Sensor Measurement Injection/Plant Model ==
  note: Change product block with you plant mode l
  note: Change the constant values according to the plant requirements
  Injection Strategy : Inport
  Input Signal : Inport  Port=2
  Constant : Constant  Value=0
  Constant2 : Constant  Value=2
  Product : Product
  "Switch " : Switch  Criteria=u2 > Threshold  Threshold=0.75  ZeroCross=off
  Injected Signal : Outport
  wires:
  Constant/1 -> "Switch "/3
  Injection Strategy/1 -> "Switch "/2
  Constant2/1 -> "Switch "/1
  "Switch "/1 -> Product/1
  Product/1 -> Injected Signal/1
  Input Signal/1 -> Product/2

== system FDIA_Toolbox/NMRI - Zero/Attack Injection Strategy ==
  Input : Inport
  " 1" : DataTypeConversion  OutMin=15  OutMax=16  OutDataTypeStr=uint8  ConvertRealWorld=Stored Integer (SI)  RndMeth=Round  SaturateOnIntegerOverflow=on  LockScale=on
  Bit to Integer Converter2 : commutil2/Bit to Integer Converter  nbits=32  bitOrder=MSB first  signedOutputValues=Unsigned  outDtype=uint8  outDtypeSigned=int8
  Data Type Conversion2 : DataTypeConversion  OutMin=15  OutMax=16  OutDataTypeStr=uint8  ConvertRealWorld=Stored Integer (SI)  RndMeth=Round  SaturateOnIntegerOverflow=on  LockScale=on
  Integer to Bit Converter : commutil2/Integer to Bit Converter  nbits=32  signedInputValues=Unsigned  bitOrder=MSB first  outDtype=uint8
  Subsystem : Subsystem
  Injected Signal : Outport
  wires:
  " 1"/1 -> Injected Signal/1
  Data Type Conversion2/1 -> Integer to Bit Converter/1
  Integer to Bit Converter/1 -> Subsystem/1(In1)
  Bit to Integer Converter2/1 -> " 1"/1
  Subsystem/1(Attacked) -> Bit to Integer Converter2/1
  Input/1 -> Data Type Conversion2/1

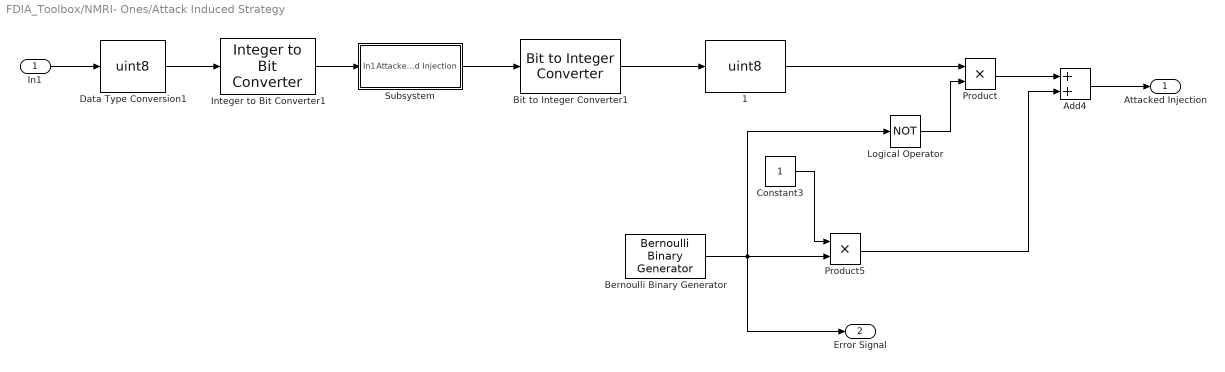
== system FDIA_Toolbox/NMRI- Ones/Attack Induced Strategy ==
  In1 : Inport
  " 1" : DataTypeConversion  OutMin=15  OutMax=16  OutDataTypeStr=uint8  ConvertRealWorld=Stored Integer (SI)  RndMeth=Round  SaturateOnIntegerOverflow=on  LockScale=on
  Add4 : Sum
  Bernoulli Binary Generator : commrandsrc3/Bernoulli Binary Generator  ProbabilityOfZero=0.9  SeedSource=Auto  Seed=0  SampleTime=1  SamplesPerFrame=1  OutputDataType=boolean  SimulateUsing=Interpreted execution
  Bit to Integer Converter1 : commutil2/Bit to Integer Converter  nbits=32  bitOrder=MSB first  signedOutputValues=Unsigned  outDtype=uint8  outDtypeSigned=int8
  Constant3 : Constant  OutDataTypeStr=boolean
  Data Type Conversion1 : DataTypeConversion  OutMin=15  OutMax=16  OutDataTypeStr=uint8  ConvertRealWorld=Stored Integer (SI)  RndMeth=Round  SaturateOnIntegerOverflow=on  LockScale=on
  Integer to Bit Converter1 : commutil2/Integer to Bit Converter  nbits=32  signedInputValues=Unsigned  bitOrder=MSB first  outDtype=uint8
  Logical Operator : Logic  Operator=NOT  AllPortsSameDT=off  OutDataTypeStr=boolean
  Product : Product  OutDataTypeStr=uint8
  Product5 : Product  OutDataTypeStr=uint8
  Subsystem : Subsystem
  Attacked Injection : Outport
  Error Signal : Outport  Port=2
  wires:
  In1/1 -> Data Type Conversion1/1
  Bernoulli Binary Generator/1 -> Error Signal/1, Logical Operator/1, Product5/2
  Bit to Integer Converter1/1 -> " 1"/1
  Subsystem/1(Attacked Injection) -> Bit to Integer Converter1/1
  Integer to Bit Converter1/1 -> Subsystem/1(In1)
  Data Type Conversion1/1 -> Integer to Bit Converter1/1
  Constant3/1 -> Product5/1
  " 1"/1 -> Product/1
  Logical Operator/1 -> Product/2
  Add4/1 -> Attacked Injection/1
  Product/1 -> Add4/1
  Product5/1 -> Add4/2

== system FDIA_Toolbox/  /Attack Induced System/Subsystem ==
  In1 : Inport
  Demux : Demux
  Mux : Mux
  Saturation{,1..3} (4 alike) : Saturate  UpperLimit=1  LowerLimit=0
  Attacked Injection : Outport
  wires:
  Demux/3 -> Saturation2/1
  Demux/2 -> Saturation1/1
  In1/1 -> Demux/1
  Mux/1 -> Attacked Injection/1
  Demux/1 -> Saturation/1
  Demux/4 -> Saturation3/1
  Saturation/1 -> Mux/1
  Saturation3/1 -> Mux/4
  Saturation2/1 -> Mux/3
  Saturation1/1 -> Mux/2

== system FDIA_Toolbox/  /Attack Induced System1/tank  ==
  flow in : Inport
  flow in1 : Inport  Port=2
  1/area : Gain  Gain=1/area  SaturateOnIntegerOverflow=on  OutDataTypeStr=Inherit: Same as input  ParamDataTypeStr=Inherit: Same as input
  Overflow sensor : Relay  OnSwitchValue=1  OffSwitchValue=0  OnOutputValue=3  ZeroCross=off
  outletArea : Gain  Gain=outletArea  SaturateOnIntegerOverflow=on  OutDataTypeStr=Inherit: Same as input  ParamDataTypeStr=Inherit: Same as input
  sqrt(2gh) : Fcn  Expr=sqrt(2*9.8*u)
  sum : Sum  Inputs=+-  SaturateOnIntegerOverflow=on  InputSameDT=on  OutDataTypeStr=Inherit: Same as first input
  tank volume : Subsystem  mask(Limited integrator.){lb=0, ub=ht * area, xi=initialHt * area}
      mask prompts: lb "Lower bound:"; ub "Upper bound:"; xi "Initial condition"
      mask help: Limited integrator
      mask Help: Implements a limited integrator with \nan expression of the form:\n\nif(x<=lb and u<0) or (x>=ub and u>0)\n\txdot=0\nelse\n\txdot=u.
      mask Display: plot(-1,-0.2,3.5,1.2,[0.05,1,2,2.9],[0,0,1,1]);disp(' 1/s    ')
  water level : Outport  InitialOutput=0
  flow out : Outport  Port=2  InitialOutput=0
  overflow flag : Outport  Port=3  InitialOutput=0
  water level1 : Outport  Port=4  InitialOutput=0
  wires:
  outletArea/1 -> flow out/1, sum/2
  sqrt(2gh)/1 -> outletArea/1
  1/area/1 -> water level1/1, sqrt(2gh)/1
  tank volume/1(Out_1) -> 1/area/1
  Overflow sensor/1 -> overflow flag/1
  flow in/1 -> sum/1
  sum/1 -> tank volume/1(In_1)
  flow in1/1 -> water level/1, Overflow sensor/1

== system FDIA_Toolbox/  /Attack Induced System1/valve ==
  control : Inport
  source flow : Inport  Port=2
  Limited Integrator : Subsystem  mask(Limited integrator.){lb=0, ub=1, xi=InitialPosition}
      mask prompts: lb "Lower bound:"; ub "Upper bound:"; xi "Initial condition"
      mask help: Limited integrator
      mask Help: Implements a limited integrator with \nan expression of the form:\n\nif(x<=lb and u<0) or (x>=ub and u>0)\n\txdot=0\nelse\n\txdot=u.
      mask Display: plot(-1,-0.2,3.5,1.2,[0.05,1,2,2.9],[0,0,1,1]);disp(' 1/s    ')
  Product : Product  SaturateOnIntegerOverflow=on  RndMeth=Zero  InputSameDT=on  OutDataTypeStr=Inherit: Same as first input
  out flow : Outport  InitialOutput=0
  wires:
  source flow/1 -> Product/2
  Product/1 -> out flow/1
  control/1 -> Limited Integrator/1(In_1)
  Limited Integrator/1(Out_1) -> Product/1

== system FDIA_Toolbox/  /Attack Injected System/tank  ==
  flow in : Inport
  1/area : Gain  Gain=1/area  SaturateOnIntegerOverflow=on  OutDataTypeStr=Inherit: Same as input  ParamDataTypeStr=Inherit: Same as input
  Overflow sensor1 : Relay  OnSwitchValue=ht - overflowLimit  OffSwitchValue=ht - overflowLimit  OnOutputValue=3  ZeroCross=off
  outletArea : Gain  Gain=outletArea  SaturateOnIntegerOverflow=on  OutDataTypeStr=Inherit: Same as input  ParamDataTypeStr=Inherit: Same as input
  sqrt(2gh) : Fcn  Expr=sqrt(2*9.8*u)
  sum : Sum  Inputs=+-  SaturateOnIntegerOverflow=on  InputSameDT=on  OutDataTypeStr=Inherit: Same as first input
  tank volume : Subsystem  mask(Limited integrator.){lb=0, ub=ht * area, xi=initialHt * area}
      mask prompts: lb "Lower bound:"; ub "Upper bound:"; xi "Initial condition"
      mask help: Limited integrator
      mask Help: Implements a limited integrator with \nan expression of the form:\n\nif(x<=lb and u<0) or (x>=ub and u>0)\n\txdot=0\nelse\n\txdot=u.
      mask Display: plot(-1,-0.2,3.5,1.2,[0.05,1,2,2.9],[0,0,1,1]);disp(' 1/s    ')
  water level : Outport  InitialOutput=0
  flow out : Outport  Port=2  InitialOutput=0
  overflow flag1 : Outport  Port=3  InitialOutput=0
  wires:
  outletArea/1 -> sum/2, flow out/1
  sqrt(2gh)/1 -> outletArea/1
  tank volume/1(Out_1) -> 1/area/1
  flow in/1 -> sum/1
  sum/1 -> tank volume/1(In_1)
  Overflow sensor1/1 -> overflow flag1/1
  1/area/1 -> sqrt(2gh)/1, Overflow sensor1/1, water level/1

== system FDIA_Toolbox/  /Attack Injected System/valve ==
  control : Inport
  source flow : Inport  Port=2
  Limited Integrator : Subsystem  mask(Limited integrator.){lb=0, ub=1, xi=InitialPosition}
      mask prompts: lb "Lower bound:"; ub "Upper bound:"; xi "Initial condition"
      mask help: Limited integrator
      mask Help: Implements a limited integrator with \nan expression of the form:\n\nif(x<=lb and u<0) or (x>=ub and u>0)\n\txdot=0\nelse\n\txdot=u.
      mask Display: plot(-1,-0.2,3.5,1.2,[0.05,1,2,2.9],[0,0,1,1]);disp(' 1/s    ')
  Product : Product  SaturateOnIntegerOverflow=on  RndMeth=Zero  InputSameDT=on  OutDataTypeStr=Inherit: Same as first input
  out flow : Outport  InitialOutput=0
  wires:
  source flow/1 -> Product/2
  Product/1 -> out flow/1
  control/1 -> Limited Integrator/1(In_1)
  Limited Integrator/1(Out_1) -> Product/1

== system FDIA_Toolbox/  /Attack Injected System1/Manual Signal ==
  In1 : Inport
  Add1 : Sum  Inputs=+-
  Add3 : Sum
  Continuous-Time VCO : commsynccomp2/Continuous-Time VCO  Ac=0.1  Fc=5  Kc=1  Ph=0
      settings: SourceProductName=Communications System Toolbox  SourceProductBaseCode=CM
  Repeating Sequence Stair : simulink/Sources/Repeating Sequence Stair  OutValues=[0.9 1 1 0.9].'  tsamp=2  OutMin=[]  OutMax=[]  OutDataTypeStr=double  OutputDataTypeScalingMode=double  OutDataType=fixdt(0,8)  ConRadixGroup=Best Precision: Vector-wise  OutScaling=2^-12
  Sine Wave1 : Sin  SineType=Sample based  Amplitude=0.1  Frequency=10  Samples=1000  SampleTime=0.01
  Out1 : Outport
  wires:
  Add3/1 -> Add1/1
  Repeating Sequence Stair/1 -> Add3/1
  Sine Wave1/1 -> Continuous-Time VCO/1
  Continuous-Time VCO/1 -> Add3/2
  Add1/1 -> Out1/1
  In1/1 -> Add1/2

== system FDIA_Toolbox/  /Attack Injected System2/Original System ==
  Constant1 : Constant  Value=0
  Constant4 : Constant  Value=2
  Constant5 : Constant
  Pulse Generator3 : DiscretePulseGenerator  PulseType=Time based  Amplitude=2  Period=10  PulseWidth=70
  Scope1 : Scope  NumInputPorts=3
  motor 1 : Switch  Criteria=u2 > Threshold  Threshold=0.75  ZeroCross=off
  tank 1 : Subsystem  mask(Water tank){ht=15, area=1, outletArea=0.1, overflowLimit=0, initialHt=0}
      mask prompts: ht "Height of tank (m):"; area "Bottom area (m^2):"; outletArea "Out pipe crossection (m^2):"; overflowLimit "Overflow sensor distance from top (m):"; initialHt "Initial level height (m):"
      mask help: Cylindrical water tank with overflow signal
      mask Display: disp('WATER\nTANK')
  valve1 : Subsystem  mask(Valve){InitialPosition=0}
      mask prompts: InitialPosition "Initial position [0=closed 1=open]:"
      mask help: Valve
      mask Display: disp('VALVE')
  Out1 : Outport
  wires:
  tank 1/2(flow out) -> Scope1/2
  Constant5/1 -> valve1/1(control)
  Constant1/1 -> motor 1/3
  motor 1/1 -> valve1/2(source flow)
  Constant4/1 -> motor 1/1
  tank 1/1(water level) -> Out1/1, Scope1/1
  Pulse Generator3/1 -> motor 1/2
  valve1/1(out flow) -> tank 1/1(flow in)
  tank 1/3(overflow flag1) -> Scope1/3

== system FDIA_Toolbox/  /Attack Injected System2/tank  ==
  flow in : Inport
  1/area : Gain  Gain=1/area  SaturateOnIntegerOverflow=on  OutDataTypeStr=Inherit: Same as input  ParamDataTypeStr=Inherit: Same as input
  Overflow sensor1 : Relay  OnSwitchValue=ht - overflowLimit  OffSwitchValue=ht - overflowLimit  OnOutputValue=3  ZeroCross=off
  outletArea : Gain  Gain=outletArea  SaturateOnIntegerOverflow=on  OutDataTypeStr=Inherit: Same as input  ParamDataTypeStr=Inherit: Same as input
  sqrt(2gh) : Fcn  Expr=sqrt(2*9.8*u)
  sum : Sum  Inputs=+-  SaturateOnIntegerOverflow=on  InputSameDT=on  OutDataTypeStr=Inherit: Same as first input
  tank volume : Subsystem  mask(Limited integrator.){lb=0, ub=ht * area, xi=initialHt * area}
      mask prompts: lb "Lower bound:"; ub "Upper bound:"; xi "Initial condition"
      mask help: Limited integrator
      mask Help: Implements a limited integrator with \nan expression of the form:\n\nif(x<=lb and u<0) or (x>=ub and u>0)\n\txdot=0\nelse\n\txdot=u.
      mask Display: plot(-1,-0.2,3.5,1.2,[0.05,1,2,2.9],[0,0,1,1]);disp(' 1/s    ')
  water level : Outport  InitialOutput=0
  flow out : Outport  Port=2  InitialOutput=0
  overflow flag1 : Outport  Port=3  InitialOutput=0
  wires:
  outletArea/1 -> sum/2, flow out/1
  sqrt(2gh)/1 -> outletArea/1
  tank volume/1(Out_1) -> 1/area/1
  flow in/1 -> sum/1
  sum/1 -> tank volume/1(In_1)
  Overflow sensor1/1 -> overflow flag1/1
  1/area/1 -> sqrt(2gh)/1, Overflow sensor1/1, water level/1
